simulink model "Ground"  (R2017b)
settings: Solver=FixedStepDiscrete  StartTime=0.0  StopTime=10.0  FixedStep=0.100000  RelTol=1e-3  EnableMultiTasking=on
model workspace (MAT data in the model file):
  already_pp = 0
  input_struct.time = [0; 0.1; 0.2; 0.3; 0.4; 0.5; 0.6; 0.7; 0.8; 0.9; 1; 1.1; 1.2; 1.3; 1.4; 1.5; 1.6; 1.7; 1.8; 1.9; 2; 2.1; 2.2; 2.3; 2.4; 2.5; 2.6; 2.7; 2.8; 2.9; 3; 3.1; 3.2; 3.3; 3.4; 3.5; 3.6; 3.7; 3.8; 3.9; 4; 4.1; 4.2; 4.3; 4.4; 4.5; 4.6; 4.7; 4.8; 4.9; 5; 5.1; 5.2; 5.3; 5.4; 5.5; 5.6; 5.7; 5.8; 5.9; 6; 6.1; 6.2; 6.3; 6.4; 6.5; 6.6; 6.7; 6.8; 6.9; 7; 7.1; 7.2; 7.3; 7.4; 7.5; 7.6; 7.7; 7.8; 7.9; 8; 8.1; 8.2; 8.3; 8.4; 8.5; 8.6; 8.7; 8.8; 8.9; 9; 9.1; 9.2; 9.3; 9.4; 9.5; 9.6; 9.7; 9.8; 9.9]
  input_struct.signals(1).name = 'In1'
  input_struct.signals(1).values = [-68; 59; -38; 6; -67; 20; -48; 31; 38; 50; -10; -84; -54; 83; -70; 65; 8; 100; -85; -12; -79; 93; -100; 55; 64; 74; -84; -20; -48; 60; -14; 83; -64; -47; -71; -73; 74; 16; 10; -71; 71; 25; -30; 3; -20; -85; -52; -76; -64; -52; -17; -91; 81; 89; -2; -2; -33; 80; -26; -78; 56; -22; -52; -19; -81; -74; 89; 92; 15; -88; -53; -30; 65; -97; -92; -67; 30; 47; 30; -10; 9; -41; 49; -63; 38; -64; -26; 25; 56; -84; 86; 55; -3; -13; -11; -39; 2; 2; 64; 59]
  input_struct.signals(1).dimensions = 1
  input_struct.signals(2).name = 'In2'
  input_struct.signals(2).values = [28.8636260387; -24.2781234679; 62.3160916565; 6.56511775989; -29.8545792846; 87.8003124; 75.1885622986; 10.0312685797; 24.4950172002; 17.4089409063; -58.4515414534; -39.7507339441; -5.81533029648; -53.9023679577; 68.8617585391; -61.0471420866; -54.8156438055; -65.8583905704; -54.4671404367; -12.8602631792; -37.7795426699; 84.6759284206; -13.9585217341; -63.0367359752; 80.976193736; 95.9496756712; -12.2260053748; -77.7761553119; -48.3870608176; -18.2560307775; 18.9792148017; -47.5576504438; 20.5686178764; 42.2431560867; -55.6506531966; -76.5164698288; -40.6648253563; -36.2443396148; -15.1666480572; 1.57165693222; -82.896840582; -47.5035530603; 60.2029245539; -94.1559444876; 85.7708278956; 46.0661725711; -2.27820523928; 15.7050122047; -52.5432840457; -8.23023436401; 92.6177078574; 9.36114374779; 4.2271661608; -53.6811226583; -2.22045121597; 24.8120176347; 35.8271081731; -20.8969568663; -26.5126702911; 97.5964006323; -92.4522267521; 77.0336016405; 82.6573655278; 59.236774717; -80.2575442689; -47.6257632259; -32.9286320074; 35.9455902755; -72.6893725289; 44.2454997163; -78.6476276786; 30.7514697337; -1.16521267215; 55.8103446463; 43.0074156801; 80.7441121113; 78.1845008662; -33.1673894525; 39.749166467; -60.4380346628; -93.8918107391; 48.8148520735; 0.00448711804017; -4.01557177079; 80.9444476135; 21.9733296845; 23.5332779177; 71.8884611292; 61.0978849059; 15.3443031229; -63.415506117; -52.0135978863; 77.3023866152; -94.2651695072; -2.01972229756; -66.4145708635; 95.7361299282; 42.5388943358; 0.0943248309686; -5.78232509161]
  input_struct.signals(2).dimensions = 1
  input_struct.signals(3).name = 'In3'
  input_struct.signals(3).values = [0; 1; 0; 0; 1; 0; 1; 1; 1; 0; 1; 1; 1; 1; 1; 0; 0; 1; 0; 0; 0; 0; 1; 1; 0; 0; 1; 0; 1; 1; 0; 0; 0; 1; 0; 0; 0; 0; 0; 0; 1; 1; 0; 1; 0; 0; 1; 1; 0; 1; 0; 1; 1; 1; 1; 1; 0; 0; 1; 0; 0; 1; 1; 1; 0; 0; 0; 1; 0; 1; 1; 0; 0; 0; 0; 0; 1; 0; 0; 1; 0; 0; 1; 0; 1; 1; 1; 0; 1; 0; 1; 1; 1; 0; 1; 0; 0; 0; 0; 0]
  input_struct.signals(3).dimensions = 1
settings Model: Creator=ktrinh  LastModifiedBy=hbourbou
settings DataIOCC: SaveFormat=Structure
settings OptimizationCC: LifeSpan=inf
settings DebuggingCC: AlgebraicLoopMsg=error  ArtificialAlgebraicLoopMsg=error  SFUnexpectedBacktrackingDiag=warning  SFNoUnconditionalDefaultTransitionDiag=warning  SFExecutionAtInitializationDiag=none
settings HardwareCC: ProdBitPerSizeT=32  ProdBitPerPtrDiffT=32  ProdWordSize=32  ProdHWDeviceType=Specified
settings CodeAppCC: StateflowObjectComments=on
settings GRTTargetCC: TargetLangStandard=C89/C90 (ANSI)  GeneratePreprocessorConditionals=Disable all
settings ConfigComp: CovMetricSettings=dw  CovHtmlReporting=on  CovSaveCumulativeToWorkspaceVar=on  CovSaveSingleToWorkspaceVar=on  CovExternalEMLEnable=off

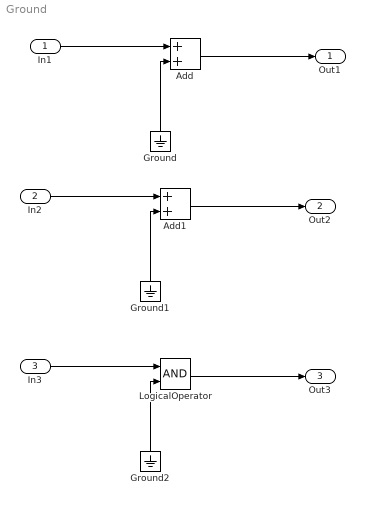
== system Ground ==
  In1 : Inport  OutDataTypeStr=int8  PortDimensions=1  SampleTime=0.1
  In2 : Inport  Port=2  OutDataTypeStr=double  PortDimensions=1  SampleTime=0.1
  In3 : Inport  Port=3  OutDataTypeStr=boolean  PortDimensions=1  SampleTime=0.1
  Add : Sum
  Add1 : Sum
  Ground : Ground
  Ground1 : Ground
  Ground2 : Ground
  LogicalOperator : Logic  AllPortsSameDT=off  OutDataTypeStr=boolean
  Out1 : Outport
  Out2 : Outport  Port=2
  Out3 : Outport  Port=3
  wires:
  In1/1 -> Add/1
  Add/1 -> Out1/1
  Ground/1 -> Add/2
  Ground1/1 -> Add1/2
  Add1/1 -> Out2/1
  In2/1 -> Add1/1
  Ground2/1 -> LogicalOperator/2
  LogicalOperator/1 -> Out3/1
  In3/1 -> LogicalOperator/1
